simulink model "LUT_liver_pancreas_35"  (R2023b)
settings: Solver=FixedStepAuto  StartTime=0  StopTime=10.1  FixedStep=Timegap  RelTol=1e-3
model workspace (MAT data in the model file):
  T1_input = 1.34
(part 1 of 3)
settings Model: Creator=ppxmr2  LastModifiedBy=ppxmr2

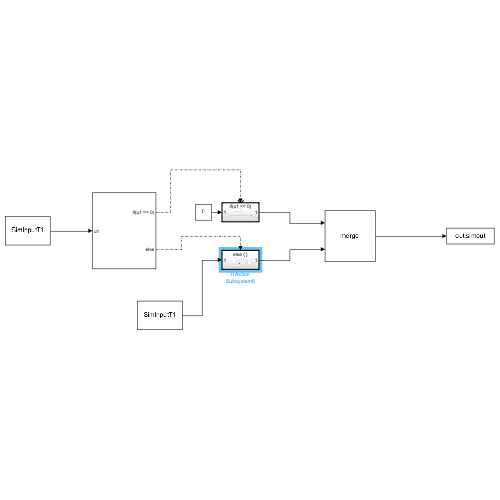
[thumbnail: Simulink's stored preview of the top-level diagram]
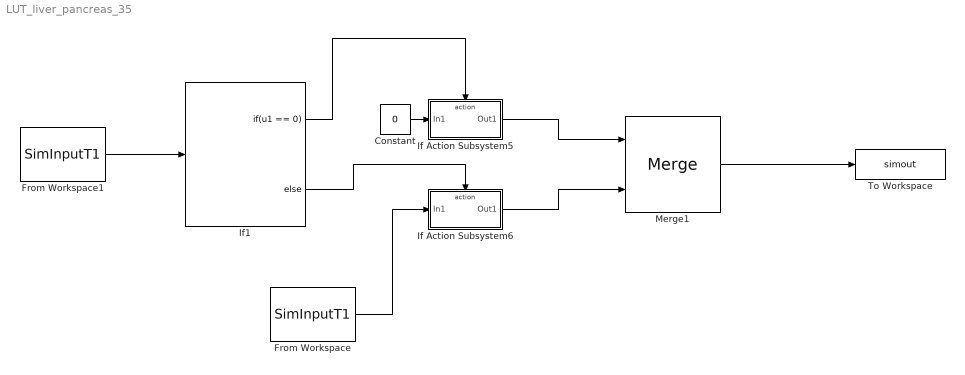
== system LUT_liver_pancreas_35 ==
  Constant : Constant  Value=0
  From Workspace : FromWorkspace  VariableName=SimInputT1  Interpolate=off  OutputAfterFinalValue=Setting to zero
  From Workspace1 : FromWorkspace  VariableName=SimInputT1  Interpolate=off  OutputAfterFinalValue=Setting to zero
  If Action Subsystem5 : Subsystem  TreatAsAtomicUnit=on
  If Action Subsystem6 : Subsystem  TreatAsAtomicUnit=on
  If1 : If  IfExpression=u1 == 0
  Merge1 : Merge
  To Workspace : ToWorkspace  VariableName=simout
  wires:
  From Workspace1/1 -> If1/1
  If1/1 -> If Action Subsystem5/Action
  If1/2 -> If Action Subsystem6/Action
  Constant/1 -> If Action Subsystem5/1(In1)
  If Action Subsystem5/1(Out1) -> Merge1/1
  If Action Subsystem6/1(Out1) -> Merge1/2
  Merge1/1 -> To Workspace/1
  From Workspace/1 -> If Action Subsystem6/1(In1)

== system LUT_liver_pancreas_35/If Action Subsystem5 ==
  In1 : Inport
  Action Port : ActionPort  ActionPortLabel=if(u1 == 0)
  Out1 : Outport
  wires:
  In1/1 -> Out1/1

== system LUT_liver_pancreas_35/If Action Subsystem6 ==
  In1 : Inport
  Action Port : ActionPort  ActionPortLabel=else
  From Workspace1 : FromWorkspace  VariableName=SimInputHR  Interpolate=off  OutputAfterFinalValue=Setting to zero
  If : If  IfExpression=u1 >= 1.495  ElseIfExpressions=u1 >= 0.995
  If Action Subsystem1 : Subsystem  TreatAsAtomicUnit=on
  If Action Subsystem2 : Subsystem  TreatAsAtomicUnit=on
  If Action Subsystem3 : Subsystem  TreatAsAtomicUnit=on
  Merge : Merge  Inputs=3
  Out1 : Outport
  wires:
  Merge/1 -> Out1/1
  From Workspace1/1 -> If/1
  If Action Subsystem1/1(Out1) -> Merge/2
  If Action Subsystem3/1(Out1) -> Merge/3
  In1/1 -> If Action Subsystem2/1(In1), If Action Subsystem1/1(In1), If Action Subsystem3/1(In1)
  If/1 -> If Action Subsystem2/Action
  If/2 -> If Action Subsystem1/Action
  If/3 -> If Action Subsystem3/Action
  If Action Subsystem2/1(Out1) -> Merge/1

== system LUT_liver_pancreas_35/If Action Subsystem6/If Action Subsystem1 ==
  In1 : Inport
  Action Port : ActionPort  ActionPortLabel=elseif(u1 >= 0.995)
  From Workspace2 : FromWorkspace  VariableName=SimInputHR  Interpolate=off  OutputAfterFinalValue=Setting to zero
  If Action Subsystem5 : Subsystem  TreatAsAtomicUnit=on
  If Action Subsystem6 : Subsystem  TreatAsAtomicUnit=on
  If Action Subsystem7 : Subsystem  TreatAsAtomicUnit=on
  If Action Subsystem8 : Subsystem  TreatAsAtomicUnit=on
  If Action Subsystem9 : Subsystem  TreatAsAtomicUnit=on
  If1 : If  IfExpression=u1 >= 1.395  ElseIfExpressions=u1 >= 1.295, u1 >= 1.195, u1 >= 1.095
  Merge1 : Merge  Inputs=5
  Out1 : Outport
  wires:
  In1/1 -> If Action Subsystem7/1(In2), If Action Subsystem8/1(In1), If Action Subsystem9/1(In1), If Action Subsystem5/1(In1), If Action Subsystem6/1(In1)
  From Workspace2/1 -> If1/1
  If Action Subsystem9/1(Out1) -> Merge1/1
  If Action Subsystem6/1(Out1) -> Merge1/5
  If Action Subsystem8/1(Out1) -> Merge1/2
  If Action Subsystem5/1(Out1) -> Merge1/4
  If1/4 -> If Action Subsystem5/Action
  If1/2 -> If Action Subsystem8/Action
  If1/3 -> If Action Subsystem7/Action
  If Action Subsystem7/1(Out2) -> Merge1/3
  If1/5 -> If Action Subsystem6/Action
  If1/1 -> If Action Subsystem9/Action
  Merge1/1 -> Out1/1

== system LUT_liver_pancreas_35/If Action Subsystem6/If Action Subsystem2 ==
  In1 : Inport
  Action Port : ActionPort  ActionPortLabel=if(u1 >= 1.495)
  From Workspace2 : FromWorkspace  VariableName=SimInputHR  Interpolate=off  OutputAfterFinalValue=Setting to zero
  If Action Subsystem5 : Subsystem  TreatAsAtomicUnit=on
  If Action Subsystem6 : Subsystem  TreatAsAtomicUnit=on
  If Action Subsystem7 : Subsystem  TreatAsAtomicUnit=on
  If Action Subsystem8 : Subsystem  TreatAsAtomicUnit=on
  If Action Subsystem9 : Subsystem  TreatAsAtomicUnit=on
  If1 : If  IfExpression=u1 >= 1.895  ElseIfExpressions=u1 >= 1.795, u1 >= 1.695, u1 >= 1.595
  Merge1 : Merge  Inputs=5
  Out1 : Outport
  wires:
  In1/1 -> If Action Subsystem9/1(In1), If Action Subsystem8/1(In1), If Action Subsystem7/1(In1), If Action Subsystem5/1(In1), If Action Subsystem6/1(In1)
  From Workspace2/1 -> If1/1
  If Action Subsystem9/1(Out1) -> Merge1/1
  If1/4 -> If Action Subsystem5/Action
  If1/2 -> If Action Subsystem8/Action
  If1/3 -> If Action Subsystem7/Action
  If1/5 -> If Action Subsystem6/Action
  If1/1 -> If Action Subsystem9/Action
  Merge1/1 -> Out1/1
  If Action Subsystem8/1(Out1) -> Merge1/2
  If Action Subsystem7/1(Out1) -> Merge1/3
  If Action Subsystem6/1(Out1) -> Merge1/5
  If Action Subsystem5/1(Out1) -> Merge1/4

== system LUT_liver_pancreas_35/If Action Subsystem6/If Action Subsystem3 ==
  In1 : Inport
  Action Port : ActionPort  ActionPortLabel=else
  From Workspace2 : FromWorkspace  VariableName=SimInputHR  Interpolate=off  OutputAfterFinalValue=Setting to zero
  If Action Subsystem5 : Subsystem  TreatAsAtomicUnit=on
  If Action Subsystem6 : Subsystem  TreatAsAtomicUnit=on
  If Action Subsystem7 : Subsystem  TreatAsAtomicUnit=on
  If Action Subsystem8 : Subsystem  TreatAsAtomicUnit=on
  If Action Subsystem9 : Subsystem  TreatAsAtomicUnit=on
  If1 : If  IfExpression=u1 >= 0.895  ElseIfExpressions=u1 >= 0.795, u1 >= 0.695, u1 >= 0595
  Merge1 : Merge  Inputs=5
  Out1 : Outport
  wires:
  In1/1 -> If Action Subsystem8/1(In1), If Action Subsystem9/1(In2), If Action Subsystem7/1(In1), If Action Subsystem5/1(In1), If Action Subsystem6/1(In1)
  From Workspace2/1 -> If1/1
  If Action Subsystem9/1(Out2) -> Merge1/1
  If Action Subsystem6/1(Out1) -> Merge1/5
  If Action Subsystem8/1(Out1) -> Merge1/2
  If Action Subsystem5/1(Out1) -> Merge1/4
  If1/4 -> If Action Subsystem5/Action
  If1/2 -> If Action Subsystem8/Action
  If1/3 -> If Action Subsystem7/Action
  If Action Subsystem7/1(Out1) -> Merge1/3
  If1/5 -> If Action Subsystem6/Action
  If1/1 -> If Action Subsystem9/Action
  Merge1/1 -> Out1/1

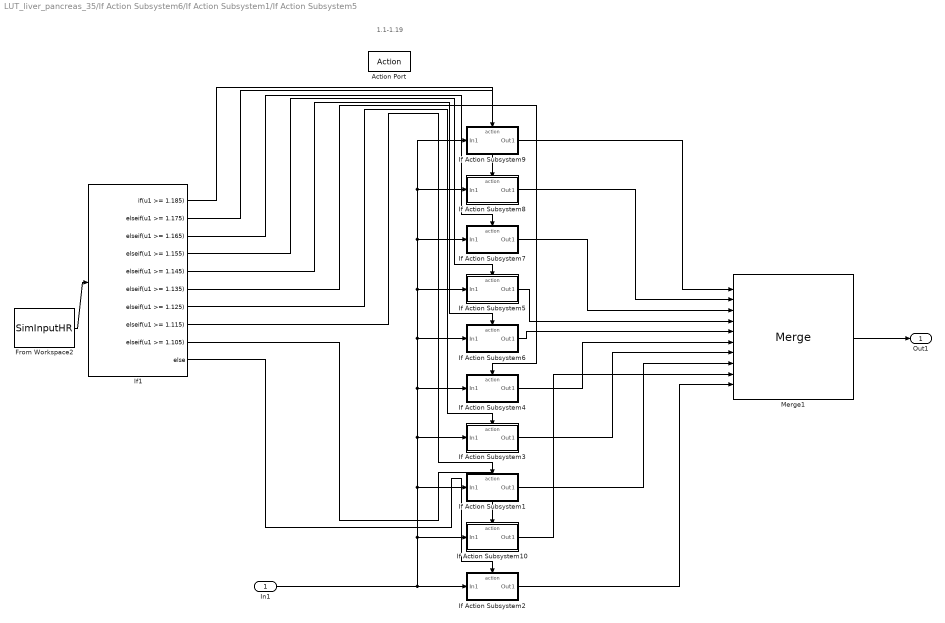
== system LUT_liver_pancreas_35/If Action Subsystem6/If Action Subsystem1/If Action Subsystem5 ==
  note: 1.1-1.19
  In1 : Inport
  Action Port : ActionPort  ActionPortLabel=elseif( u1 >= 1.095)
  From Workspace2 : FromWorkspace  VariableName=SimInputHR  Interpolate=off  OutputAfterFinalValue=Setting to zero
  If Action Subsystem1 : Subsystem  TreatAsAtomicUnit=on
  If Action Subsystem10 : Subsystem  TreatAsAtomicUnit=on
  If Action Subsystem2 : Subsystem  TreatAsAtomicUnit=on
  If Action Subsystem3 : Subsystem  TreatAsAtomicUnit=on
  If Action Subsystem4 : Subsystem  TreatAsAtomicUnit=on
  If Action Subsystem5 : Subsystem  TreatAsAtomicUnit=on
  If Action Subsystem6 : Subsystem  TreatAsAtomicUnit=on
  If Action Subsystem7 : Subsystem  TreatAsAtomicUnit=on
  If Action Subsystem8 : Subsystem  TreatAsAtomicUnit=on
  If Action Subsystem9 : Subsystem  TreatAsAtomicUnit=on
  If1 : If  IfExpression=u1 >= 1.185  ElseIfExpressions=u1 >= 1.175, u1 >= 1.165, u1 >= 1.155, u1 >= 1.145, u1 >= 1.135, u1 >= 1.125, u1 >= 1.115, u1 >= 1.105
  Merge1 : Merge  Inputs=10
  Out1 : Outport
  wires:
  If1/10 -> If Action Subsystem2/Action
  If Action Subsystem4/1(Out1) -> Merge1/6
  From Workspace2/1 -> If1/1
  If Action Subsystem6/1(Out1) -> Merge1/5
  Merge1/1 -> Out1/1
  If1/8 -> If Action Subsystem1/Action
  If Action Subsystem3/1(Out1) -> Merge1/7
  In1/1 -> If Action Subsystem1/1(In1), If Action Subsystem3/1(In1), If Action Subsystem4/1(In1), If Action Subsystem7/1(In1), If Action Subsystem8/1(In1), If Action Subsystem9/1(In1), If Action Subsystem5/1(In1), If Action Subsystem6/1(In1), If Action Subsystem10/1(In1), If Action Subsystem2/1(In1)
  If1/6 -> If Action Subsystem4/Action
  If Action Subsystem1/1(Out1) -> Merge1/8
  If1/4 -> If Action Subsystem5/Action
  If Action Subsystem8/1(Out1) -> Merge1/2
  If1/5 -> If Action Subsystem6/Action
  If Action Subsystem7/1(Out1) -> Merge1/3
  If1/3 -> If Action Subsystem7/Action
  If1/7 -> If Action Subsystem3/Action
  If Action Subsystem5/1(Out1) -> Merge1/4
  If Action Subsystem2/1(Out1) -> Merge1/10
  If1/2 -> If Action Subsystem8/Action
  If1/1 -> If Action Subsystem9/Action
  If Action Subsystem9/1(Out1) -> Merge1/1
  If1/9 -> If Action Subsystem10/Action
  If Action Subsystem10/1(Out1) -> Merge1/9

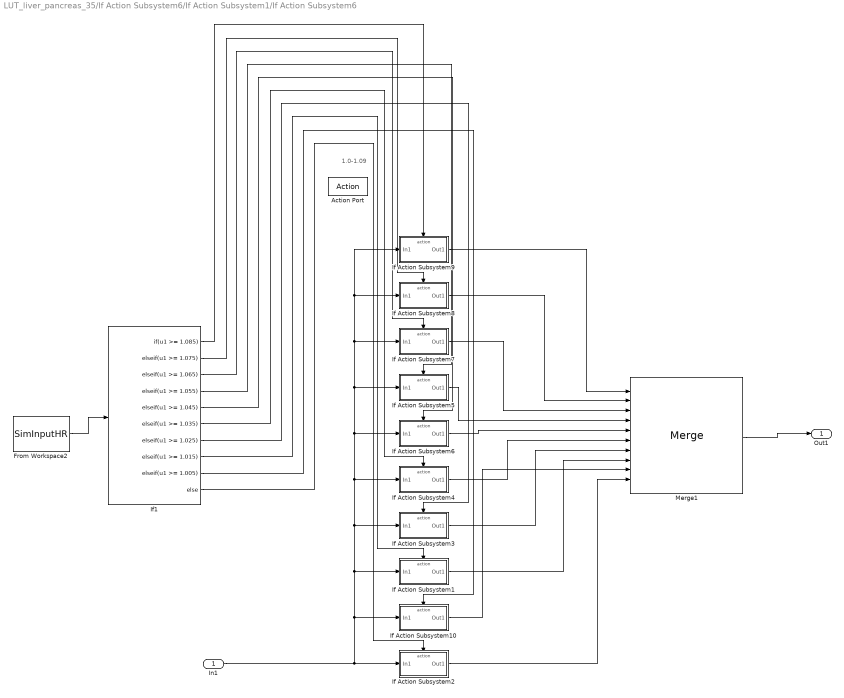
== system LUT_liver_pancreas_35/If Action Subsystem6/If Action Subsystem1/If Action Subsystem6 ==
  note: 1.0-1.09
  In1 : Inport
  Action Port : ActionPort  ActionPortLabel=else
  From Workspace2 : FromWorkspace  VariableName=SimInputHR  Interpolate=off  OutputAfterFinalValue=Setting to zero
  If Action Subsystem1 : Subsystem  TreatAsAtomicUnit=on
  If Action Subsystem10 : Subsystem  TreatAsAtomicUnit=on
  If Action Subsystem2 : Subsystem  TreatAsAtomicUnit=on
  If Action Subsystem3 : Subsystem  TreatAsAtomicUnit=on
  If Action Subsystem4 : Subsystem  TreatAsAtomicUnit=on
  If Action Subsystem5 : Subsystem  TreatAsAtomicUnit=on
  If Action Subsystem6 : Subsystem  TreatAsAtomicUnit=on
  If Action Subsystem7 : Subsystem  TreatAsAtomicUnit=on
  If Action Subsystem8 : Subsystem  TreatAsAtomicUnit=on
  If Action Subsystem9 : Subsystem  TreatAsAtomicUnit=on
  If1 : If  IfExpression=u1 >= 1.085  ElseIfExpressions=u1 >= 1.075, u1 >= 1.065, u1 >= 1.055, u1 >= 1.045, u1 >= 1.035, u1 >= 1.025, u1 >= 1.015, u1 >= 1.005
  Merge1 : Merge  Inputs=10
  Out1 : Outport
  wires:
  If1/10 -> If Action Subsystem2/Action
  If Action Subsystem4/1(Out1) -> Merge1/6
  From Workspace2/1 -> If1/1
  If Action Subsystem6/1(Out1) -> Merge1/5
  Merge1/1 -> Out1/1
  If1/8 -> If Action Subsystem1/Action
  If Action Subsystem3/1(Out1) -> Merge1/7
  In1/1 -> If Action Subsystem1/1(In1), If Action Subsystem3/1(In1), If Action Subsystem4/1(In1), If Action Subsystem7/1(In1), If Action Subsystem8/1(In1), If Action Subsystem9/1(In1), If Action Subsystem5/1(In1), If Action Subsystem6/1(In1), If Action Subsystem10/1(In1), If Action Subsystem2/1(In1)
  If1/6 -> If Action Subsystem4/Action
  If Action Subsystem1/1(Out1) -> Merge1/8
  If1/4 -> If Action Subsystem5/Action
  If Action Subsystem8/1(Out1) -> Merge1/2
  If1/5 -> If Action Subsystem6/Action
  If Action Subsystem7/1(Out1) -> Merge1/3
  If1/3 -> If Action Subsystem7/Action
  If1/7 -> If Action Subsystem3/Action
  If Action Subsystem5/1(Out1) -> Merge1/4
  If Action Subsystem2/1(Out1) -> Merge1/10
  If1/2 -> If Action Subsystem8/Action
  If1/1 -> If Action Subsystem9/Action
  If Action Subsystem9/1(Out1) -> Merge1/1
  If1/9 -> If Action Subsystem10/Action
  If Action Subsystem10/1(Out1) -> Merge1/9

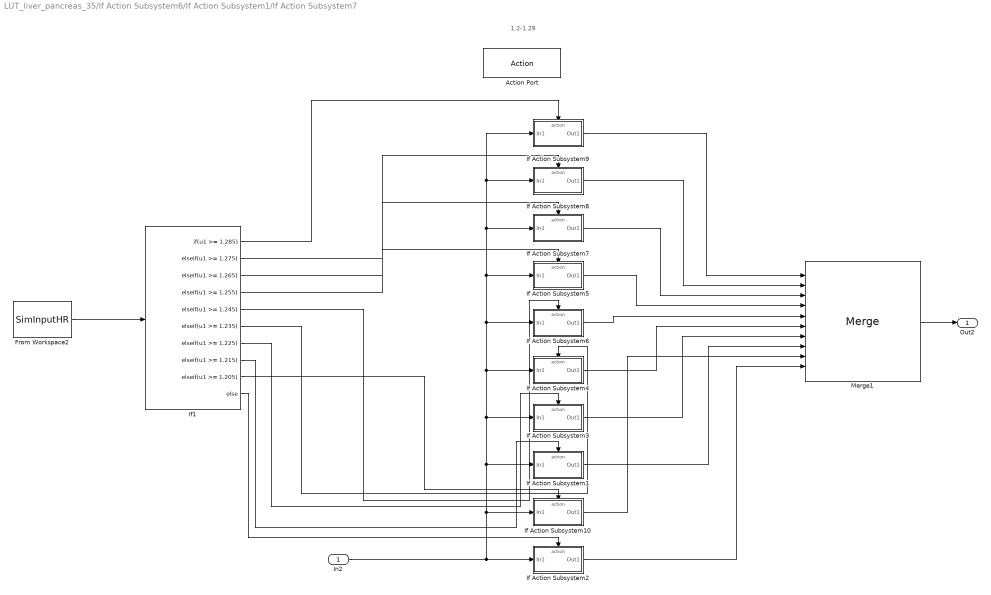
== system LUT_liver_pancreas_35/If Action Subsystem6/If Action Subsystem1/If Action Subsystem7 ==
  note: 1.2-1.29
  In2 : Inport
  Action Port : ActionPort  ActionPortLabel=elseif( u1 >= 1.195)
  From Workspace2 : FromWorkspace  VariableName=SimInputHR  Interpolate=off  OutputAfterFinalValue=Setting to zero
  If Action Subsystem1 : Subsystem  TreatAsAtomicUnit=on
  If Action Subsystem10 : Subsystem  TreatAsAtomicUnit=on
  If Action Subsystem2 : Subsystem  TreatAsAtomicUnit=on
  If Action Subsystem3 : Subsystem  TreatAsAtomicUnit=on
  If Action Subsystem4 : Subsystem  TreatAsAtomicUnit=on
  If Action Subsystem5 : Subsystem  TreatAsAtomicUnit=on
  If Action Subsystem6 : Subsystem  TreatAsAtomicUnit=on
  If Action Subsystem7 : Subsystem  TreatAsAtomicUnit=on
  If Action Subsystem8 : Subsystem  TreatAsAtomicUnit=on
  If Action Subsystem9 : Subsystem  TreatAsAtomicUnit=on
  If1 : If  IfExpression=u1 >= 1.285  ElseIfExpressions=u1 >= 1.275, u1 >= 1.265, u1 >= 1.255, u1 >= 1.245, u1 >= 1.235, u1 >= 1.225, u1 >= 1.215, u1 >= 1.205
  Merge1 : Merge  Inputs=10
  Out2 : Outport
  wires:
  If1/10 -> If Action Subsystem2/Action
  If Action Subsystem4/1(Out1) -> Merge1/6
  From Workspace2/1 -> If1/1
  If Action Subsystem6/1(Out1) -> Merge1/5
  Merge1/1 -> Out2/1
  If1/8 -> If Action Subsystem1/Action
  If Action Subsystem3/1(Out1) -> Merge1/7
  In2/1 -> If Action Subsystem1/1(In1), If Action Subsystem3/1(In1), If Action Subsystem4/1(In1), If Action Subsystem7/1(In1), If Action Subsystem8/1(In1), If Action Subsystem9/1(In1), If Action Subsystem5/1(In1), If Action Subsystem6/1(In1), If Action Subsystem10/1(In1), If Action Subsystem2/1(In1)
  If1/6 -> If Action Subsystem4/Action
  If Action Subsystem1/1(Out1) -> Merge1/8
  If1/4 -> If Action Subsystem5/Action
  If Action Subsystem8/1(Out1) -> Merge1/2
  If1/5 -> If Action Subsystem6/Action
  If Action Subsystem7/1(Out1) -> Merge1/3
  If1/3 -> If Action Subsystem7/Action
  If1/7 -> If Action Subsystem3/Action
  If Action Subsystem5/1(Out1) -> Merge1/4
  If Action Subsystem2/1(Out1) -> Merge1/10
  If1/2 -> If Action Subsystem8/Action
  If1/1 -> If Action Subsystem9/Action
  If Action Subsystem9/1(Out1) -> Merge1/1
  If Action Subsystem10/1(Out1) -> Merge1/9
  If1/9 -> If Action Subsystem10/Action

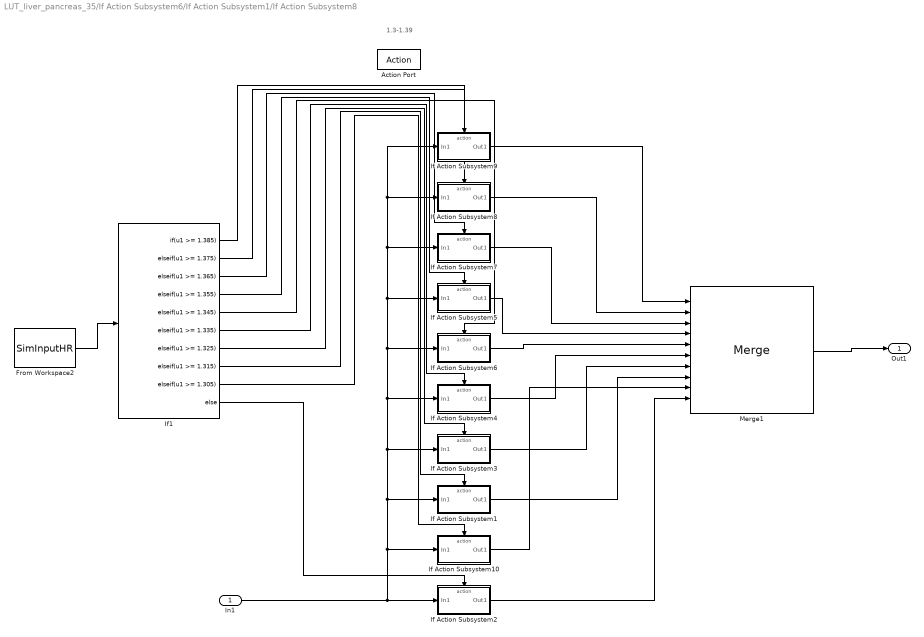
== system LUT_liver_pancreas_35/If Action Subsystem6/If Action Subsystem1/If Action Subsystem8 ==
  note: 1.3-1.39
  In1 : Inport
  Action Port : ActionPort  ActionPortLabel=elseif(u1 >= 1.295)
  From Workspace2 : FromWorkspace  VariableName=SimInputHR  Interpolate=off  OutputAfterFinalValue=Setting to zero
  If Action Subsystem1 : Subsystem  TreatAsAtomicUnit=on
  If Action Subsystem10 : Subsystem  TreatAsAtomicUnit=on
  If Action Subsystem2 : Subsystem  TreatAsAtomicUnit=on
  If Action Subsystem3 : Subsystem  TreatAsAtomicUnit=on
  If Action Subsystem4 : Subsystem  TreatAsAtomicUnit=on
  If Action Subsystem5 : Subsystem  TreatAsAtomicUnit=on
  If Action Subsystem6 : Subsystem  TreatAsAtomicUnit=on
  If Action Subsystem7 : Subsystem  TreatAsAtomicUnit=on
  If Action Subsystem8 : Subsystem  TreatAsAtomicUnit=on
  If Action Subsystem9 : Subsystem  TreatAsAtomicUnit=on
  If1 : If  IfExpression=u1 >= 1.385  ElseIfExpressions=u1 >= 1.375, u1 >= 1.365, u1 >= 1.355, u1 >= 1.345, u1 >= 1.335, u1 >= 1.325, u1 >= 1.315, u1 >= 1.305
  Merge1 : Merge  Inputs=10
  Out1 : Outport
  wires:
  If1/10 -> If Action Subsystem2/Action
  If Action Subsystem4/1(Out1) -> Merge1/6
  From Workspace2/1 -> If1/1
  If Action Subsystem6/1(Out1) -> Merge1/5
  Merge1/1 -> Out1/1
  If1/8 -> If Action Subsystem1/Action
  If Action Subsystem3/1(Out1) -> Merge1/7
  In1/1 -> If Action Subsystem1/1(In1), If Action Subsystem3/1(In1), If Action Subsystem4/1(In1), If Action Subsystem7/1(In1), If Action Subsystem8/1(In1), If Action Subsystem9/1(In1), If Action Subsystem5/1(In1), If Action Subsystem6/1(In1), If Action Subsystem10/1(In1), If Action Subsystem2/1(In1)
  If1/6 -> If Action Subsystem4/Action
  If Action Subsystem1/1(Out1) -> Merge1/8
  If1/4 -> If Action Subsystem5/Action
  If Action Subsystem8/1(Out1) -> Merge1/2
  If1/5 -> If Action Subsystem6/Action
  If Action Subsystem7/1(Out1) -> Merge1/3
  If1/3 -> If Action Subsystem7/Action
  If1/7 -> If Action Subsystem3/Action
  If Action Subsystem5/1(Out1) -> Merge1/4
  If Action Subsystem2/1(Out1) -> Merge1/10
  If1/2 -> If Action Subsystem8/Action
  If1/1 -> If Action Subsystem9/Action
  If Action Subsystem9/1(Out1) -> Merge1/1
  If1/9 -> If Action Subsystem10/Action
  If Action Subsystem10/1(Out1) -> Merge1/9

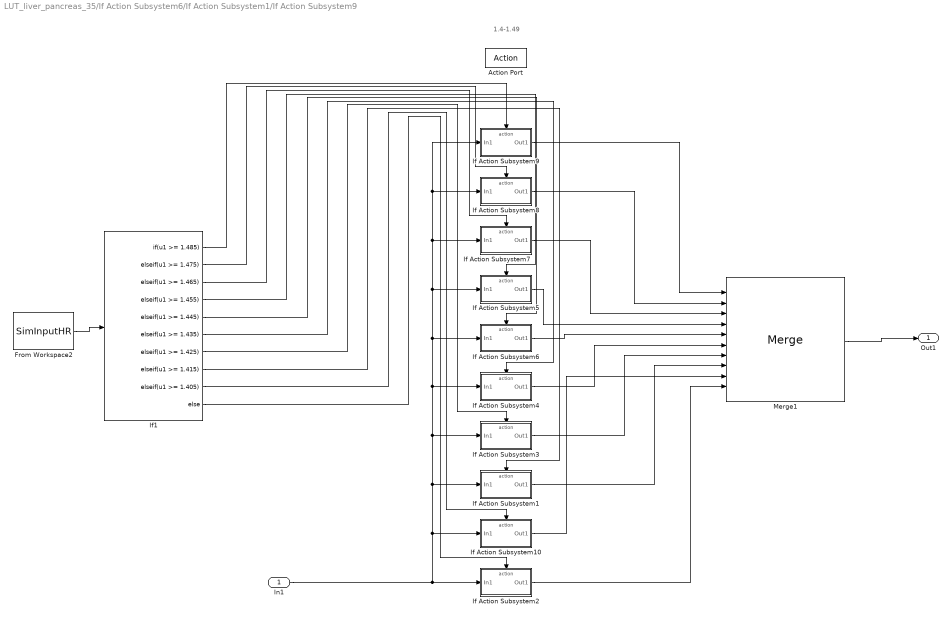
== system LUT_liver_pancreas_35/If Action Subsystem6/If Action Subsystem1/If Action Subsystem9 ==
  note: 1.4-1.49
  In1 : Inport
  Action Port : ActionPort  ActionPortLabel=if(u1 >= 1.395)
  From Workspace2 : FromWorkspace  VariableName=SimInputHR  Interpolate=off  OutputAfterFinalValue=Setting to zero
  If Action Subsystem1 : Subsystem  TreatAsAtomicUnit=on
  If Action Subsystem10 : Subsystem  TreatAsAtomicUnit=on
  If Action Subsystem2 : Subsystem  TreatAsAtomicUnit=on
  If Action Subsystem3 : Subsystem  TreatAsAtomicUnit=on
  If Action Subsystem4 : Subsystem  TreatAsAtomicUnit=on
  If Action Subsystem5 : Subsystem  TreatAsAtomicUnit=on
  If Action Subsystem6 : Subsystem  TreatAsAtomicUnit=on
  If Action Subsystem7 : Subsystem  TreatAsAtomicUnit=on
  If Action Subsystem8 : Subsystem  TreatAsAtomicUnit=on
  If Action Subsystem9 : Subsystem  TreatAsAtomicUnit=on
  If1 : If  IfExpression=u1 >= 1.485  ElseIfExpressions=u1 >= 1.475, u1 >= 1.465, u1 >= 1.455, u1 >= 1.445, u1 >= 1.435, u1 >= 1.425, u1 >= 1.415, u1 >= 1.405
  Merge1 : Merge  Inputs=10
  Out1 : Outport
  wires:
  If1/10 -> If Action Subsystem2/Action
  If Action Subsystem4/1(Out1) -> Merge1/6
  From Workspace2/1 -> If1/1
  If Action Subsystem6/1(Out1) -> Merge1/5
  Merge1/1 -> Out1/1
  If1/8 -> If Action Subsystem1/Action
  If Action Subsystem3/1(Out1) -> Merge1/7
  In1/1 -> If Action Subsystem10/1(In1), If Action Subsystem1/1(In1), If Action Subsystem3/1(In1), If Action Subsystem4/1(In1), If Action Subsystem7/1(In1), If Action Subsystem8/1(In1), If Action Subsystem9/1(In1), If Action Subsystem5/1(In1), If Action Subsystem6/1(In1), If Action Subsystem2/1(In1)
  If1/6 -> If Action Subsystem4/Action
  If Action Subsystem1/1(Out1) -> Merge1/8
  If1/4 -> If Action Subsystem5/Action
  If Action Subsystem8/1(Out1) -> Merge1/2
  If1/5 -> If Action Subsystem6/Action
  If Action Subsystem7/1(Out1) -> Merge1/3
  If1/3 -> If Action Subsystem7/Action
  If1/7 -> If Action Subsystem3/Action
  If Action Subsystem5/1(Out1) -> Merge1/4
  If Action Subsystem2/1(Out1) -> Merge1/10
  If1/2 -> If Action Subsystem8/Action
  If1/1 -> If Action Subsystem9/Action
  If Action Subsystem9/1(Out1) -> Merge1/1
  If1/9 -> If Action Subsystem10/Action
  If Action Subsystem10/1(Out1) -> Merge1/9

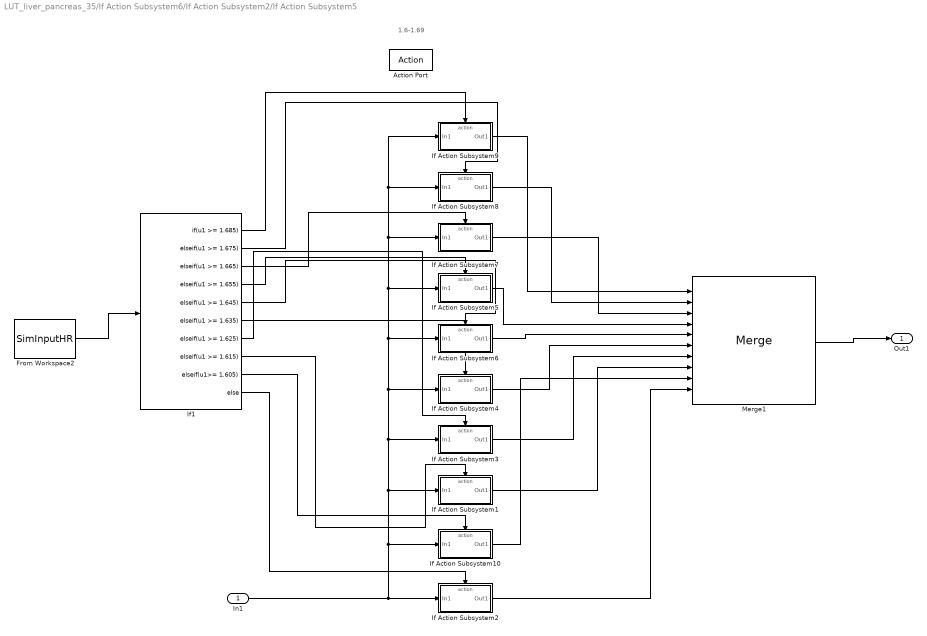
== system LUT_liver_pancreas_35/If Action Subsystem6/If Action Subsystem2/If Action Subsystem5 ==
  note: 1.6-1.69
  In1 : Inport
  Action Port : ActionPort  ActionPortLabel=elseif( u1 >= 1.595)
  From Workspace2 : FromWorkspace  VariableName=SimInputHR  Interpolate=off  OutputAfterFinalValue=Setting to zero
  If Action Subsystem1 : Subsystem  TreatAsAtomicUnit=on
  If Action Subsystem10 : Subsystem  TreatAsAtomicUnit=on
  If Action Subsystem2 : Subsystem  TreatAsAtomicUnit=on
  If Action Subsystem3 : Subsystem  TreatAsAtomicUnit=on
  If Action Subsystem4 : Subsystem  TreatAsAtomicUnit=on
  If Action Subsystem5 : Subsystem  TreatAsAtomicUnit=on
  If Action Subsystem6 : Subsystem  TreatAsAtomicUnit=on
  If Action Subsystem7 : Subsystem  TreatAsAtomicUnit=on
  If Action Subsystem8 : Subsystem  TreatAsAtomicUnit=on
  If Action Subsystem9 : Subsystem  TreatAsAtomicUnit=on
  If1 : If  IfExpression=u1 >= 1.685  ElseIfExpressions=u1 >= 1.675, u1 >= 1.665, u1 >= 1.655, u1 >= 1.645, u1 >= 1.635, u1 >= 1.625, u1 >= 1.615, u1>= 1.605
  Merge1 : Merge  Inputs=10
  Out1 : Outport
  wires:
  If1/2 -> If Action Subsystem8/Action
  If Action Subsystem5/1(Out1) -> Merge1/4
  If1/3 -> If Action Subsystem7/Action
  If Action Subsystem9/1(Out1) -> Merge1/1
  If1/7 -> If Action Subsystem3/Action
  If1/5 -> If Action Subsystem6/Action
  If1/1 -> If Action Subsystem9/Action
  If Action Subsystem4/1(Out1) -> Merge1/6
  If1/10 -> If Action Subsystem2/Action
  If Action Subsystem8/1(Out1) -> Merge1/2
  If1/4 -> If Action Subsystem5/Action
  In1/1 -> If Action Subsystem10/1(In1), If Action Subsystem1/1(In1), If Action Subsystem3/1(In1), If Action Subsystem4/1(In1), If Action Subsystem7/1(In1), If Action Subsystem8/1(In1), If Action Subsystem9/1(In1), If Action Subsystem5/1(In1), If Action Subsystem6/1(In1), If Action Subsystem2/1(In1)
  If Action Subsystem1/1(Out1) -> Merge1/8
  If Action Subsystem2/1(Out1) -> Merge1/10
  If1/8 -> If Action Subsystem1/Action
  If Action Subsystem3/1(Out1) -> Merge1/7
  If1/6 -> If Action Subsystem4/Action
  From Workspace2/1 -> If1/1
  Merge1/1 -> Out1/1
  If Action Subsystem6/1(Out1) -> Merge1/5
  If Action Subsystem7/1(Out1) -> Merge1/3
  If1/9 -> If Action Subsystem10/Action
  If Action Subsystem10/1(Out1) -> Merge1/9

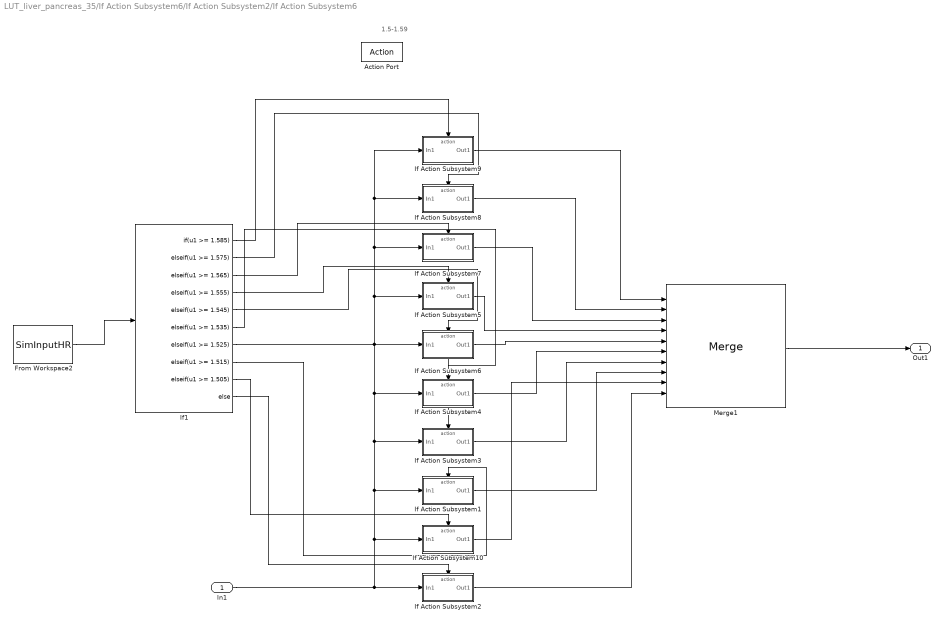
== system LUT_liver_pancreas_35/If Action Subsystem6/If Action Subsystem2/If Action Subsystem6 ==
  note: 1.5-1.59
  In1 : Inport
  Action Port : ActionPort  ActionPortLabel=else
  From Workspace2 : FromWorkspace  VariableName=SimInputHR  Interpolate=off  OutputAfterFinalValue=Setting to zero
  If Action Subsystem1 : Subsystem  TreatAsAtomicUnit=on
  If Action Subsystem10 : Subsystem  TreatAsAtomicUnit=on
  If Action Subsystem2 : Subsystem  TreatAsAtomicUnit=on
  If Action Subsystem3 : Subsystem  TreatAsAtomicUnit=on
  If Action Subsystem4 : Subsystem  TreatAsAtomicUnit=on
  If Action Subsystem5 : Subsystem  TreatAsAtomicUnit=on
  If Action Subsystem6 : Subsystem  TreatAsAtomicUnit=on
  If Action Subsystem7 : Subsystem  TreatAsAtomicUnit=on
  If Action Subsystem8 : Subsystem  TreatAsAtomicUnit=on
  If Action Subsystem9 : Subsystem  TreatAsAtomicUnit=on
  If1 : If  IfExpression=u1 >= 1.585  ElseIfExpressions=u1 >= 1.575, u1 >= 1.565, u1 >= 1.555, u1 >= 1.545, u1 >= 1.535, u1 >= 1.525, u1 >= 1.515, u1 >= 1.505
  Merge1 : Merge  Inputs=10
  Out1 : Outport
  wires:
  If1/2 -> If Action Subsystem8/Action
  If Action Subsystem5/1(Out1) -> Merge1/4
  If1/3 -> If Action Subsystem7/Action
  If Action Subsystem9/1(Out1) -> Merge1/1
  If1/7 -> If Action Subsystem3/Action
  If1/5 -> If Action Subsystem6/Action
  If1/1 -> If Action Subsystem9/Action
  If Action Subsystem4/1(Out1) -> Merge1/6
  If1/10 -> If Action Subsystem2/Action
  If Action Subsystem8/1(Out1) -> Merge1/2
  If1/4 -> If Action Subsystem5/Action
  In1/1 -> If Action Subsystem10/1(In1), If Action Subsystem1/1(In1), If Action Subsystem3/1(In1), If Action Subsystem4/1(In1), If Action Subsystem7/1(In1), If Action Subsystem8/1(In1), If Action Subsystem9/1(In1), If Action Subsystem5/1(In1), If Action Subsystem6/1(In1), If Action Subsystem2/1(In1)
  If Action Subsystem1/1(Out1) -> Merge1/8
  If Action Subsystem2/1(Out1) -> Merge1/10
  If1/8 -> If Action Subsystem1/Action
  If Action Subsystem3/1(Out1) -> Merge1/7
  If1/6 -> If Action Subsystem4/Action
  From Workspace2/1 -> If1/1
  Merge1/1 -> Out1/1
  If Action Subsystem6/1(Out1) -> Merge1/5
  If Action Subsystem7/1(Out1) -> Merge1/3
  If1/9 -> If Action Subsystem10/Action
  If Action Subsystem10/1(Out1) -> Merge1/9

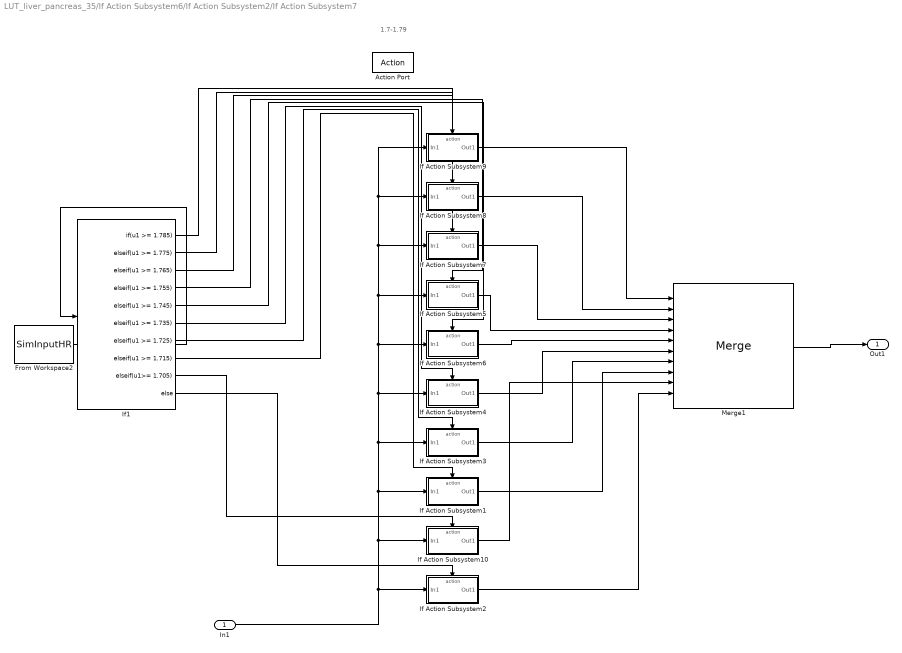
== system LUT_liver_pancreas_35/If Action Subsystem6/If Action Subsystem2/If Action Subsystem7 ==
  note: 1.7-1.79
  In1 : Inport
  Action Port : ActionPort  ActionPortLabel=elseif( u1 >= 1.695)
  From Workspace2 : FromWorkspace  VariableName=SimInputHR  Interpolate=off  OutputAfterFinalValue=Setting to zero
  If Action Subsystem1 : Subsystem  TreatAsAtomicUnit=on
  If Action Subsystem10 : Subsystem  TreatAsAtomicUnit=on
  If Action Subsystem2 : Subsystem  TreatAsAtomicUnit=on
  If Action Subsystem3 : Subsystem  TreatAsAtomicUnit=on
  If Action Subsystem4 : Subsystem  TreatAsAtomicUnit=on
  If Action Subsystem5 : Subsystem  TreatAsAtomicUnit=on
  If Action Subsystem6 : Subsystem  TreatAsAtomicUnit=on
  If Action Subsystem7 : Subsystem  TreatAsAtomicUnit=on
  If Action Subsystem8 : Subsystem  TreatAsAtomicUnit=on
  If Action Subsystem9 : Subsystem  TreatAsAtomicUnit=on
  If1 : If  IfExpression=u1 >= 1.785  ElseIfExpressions=u1 >= 1.775, u1 >= 1.765, u1 >= 1.755, u1 >= 1.745, u1 >= 1.735, u1 >= 1.725, u1 >= 1.715, u1>= 1.705
  Merge1 : Merge  Inputs=10
  Out1 : Outport
  wires:
  If1/2 -> If Action Subsystem8/Action
  If Action Subsystem5/1(Out1) -> Merge1/4
  If1/3 -> If Action Subsystem7/Action
  If Action Subsystem9/1(Out1) -> Merge1/1
  If1/7 -> If Action Subsystem3/Action
  If1/5 -> If Action Subsystem6/Action
  If1/1 -> If Action Subsystem9/Action
  If Action Subsystem4/1(Out1) -> Merge1/6
  If1/10 -> If Action Subsystem2/Action
  If Action Subsystem8/1(Out1) -> Merge1/2
  If1/4 -> If Action Subsystem5/Action
  In1/1 -> If Action Subsystem10/1(In1), If Action Subsystem1/1(In1), If Action Subsystem3/1(In1), If Action Subsystem4/1(In1), If Action Subsystem7/1(In1), If Action Subsystem8/1(In1), If Action Subsystem9/1(In1), If Action Subsystem5/1(In1), If Action Subsystem6/1(In1), If Action Subsystem2/1(In1)
  If Action Subsystem1/1(Out1) -> Merge1/8
  If Action Subsystem2/1(Out1) -> Merge1/10
  If1/8 -> If Action Subsystem1/Action
  If Action Subsystem3/1(Out1) -> Merge1/7
  If1/6 -> If Action Subsystem4/Action
  From Workspace2/1 -> If1/1
  Merge1/1 -> Out1/1
  If Action Subsystem6/1(Out1) -> Merge1/5
  If Action Subsystem7/1(Out1) -> Merge1/3
  If Action Subsystem10/1(Out1) -> Merge1/9
  If1/9 -> If Action Subsystem10/Action

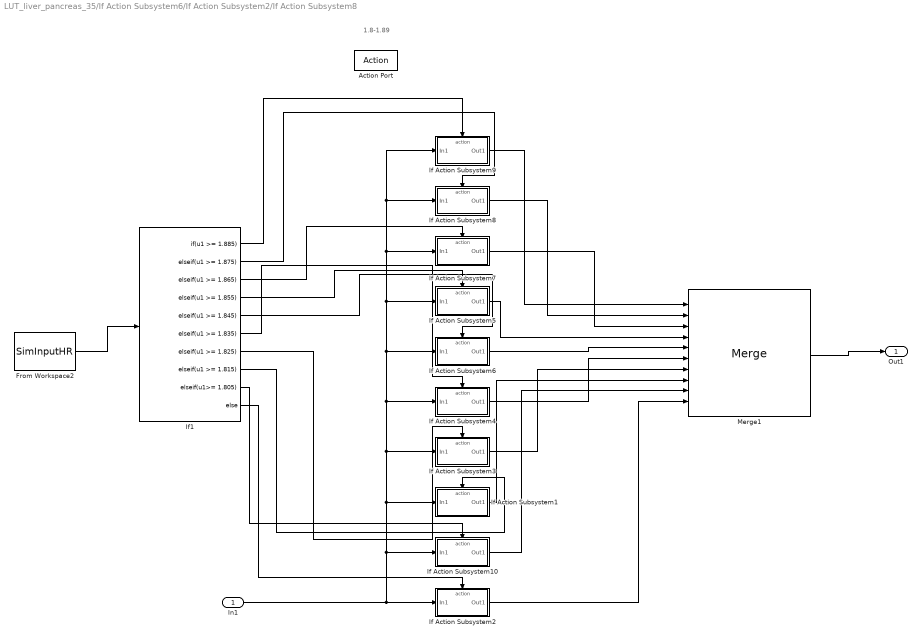
== system LUT_liver_pancreas_35/If Action Subsystem6/If Action Subsystem2/If Action Subsystem8 ==
  note: 1.8-1.89
  In1 : Inport
  Action Port : ActionPort  ActionPortLabel=elseif(u1 >= 1.795)
  From Workspace2 : FromWorkspace  VariableName=SimInputHR  Interpolate=off  OutputAfterFinalValue=Setting to zero
  If Action Subsystem1 : Subsystem  TreatAsAtomicUnit=on
  If Action Subsystem10 : Subsystem  TreatAsAtomicUnit=on
  If Action Subsystem2 : Subsystem  TreatAsAtomicUnit=on
  If Action Subsystem3 : Subsystem  TreatAsAtomicUnit=on
  If Action Subsystem4 : Subsystem  TreatAsAtomicUnit=on
  If Action Subsystem5 : Subsystem  TreatAsAtomicUnit=on
  If Action Subsystem6 : Subsystem  TreatAsAtomicUnit=on
  If Action Subsystem7 : Subsystem  TreatAsAtomicUnit=on
  If Action Subsystem8 : Subsystem  TreatAsAtomicUnit=on
  If Action Subsystem9 : Subsystem  TreatAsAtomicUnit=on
  If1 : If  IfExpression=u1 >= 1.885  ElseIfExpressions=u1 >= 1.875, u1 >= 1.865, u1 >= 1.855, u1 >= 1.845, u1 >= 1.835, u1 >= 1.825, u1 >= 1.815, u1>= 1.805
  Merge1 : Merge  Inputs=10
  Out1 : Outport
  wires:
  If1/2 -> If Action Subsystem8/Action
  If Action Subsystem5/1(Out1) -> Merge1/4
  If1/3 -> If Action Subsystem7/Action
  If Action Subsystem9/1(Out1) -> Merge1/1
  If1/7 -> If Action Subsystem3/Action
  If1/5 -> If Action Subsystem6/Action
  If1/1 -> If Action Subsystem9/Action
  If Action Subsystem4/1(Out1) -> Merge1/6
  If1/10 -> If Action Subsystem2/Action
  If Action Subsystem8/1(Out1) -> Merge1/2
  If1/4 -> If Action Subsystem5/Action
  In1/1 -> If Action Subsystem10/1(In1), If Action Subsystem1/1(In1), If Action Subsystem3/1(In1), If Action Subsystem4/1(In1), If Action Subsystem7/1(In1), If Action Subsystem8/1(In1), If Action Subsystem9/1(In1), If Action Subsystem5/1(In1), If Action Subsystem6/1(In1), If Action Subsystem2/1(In1)
  If Action Subsystem1/1(Out1) -> Merge1/8
  If Action Subsystem2/1(Out1) -> Merge1/10
  If1/8 -> If Action Subsystem1/Action
  If Action Subsystem3/1(Out1) -> Merge1/7
  If1/6 -> If Action Subsystem4/Action
  From Workspace2/1 -> If1/1
  Merge1/1 -> Out1/1
  If Action Subsystem6/1(Out1) -> Merge1/5
  If Action Subsystem7/1(Out1) -> Merge1/3
  If1/9 -> If Action Subsystem10/Action
  If Action Subsystem10/1(Out1) -> Merge1/9

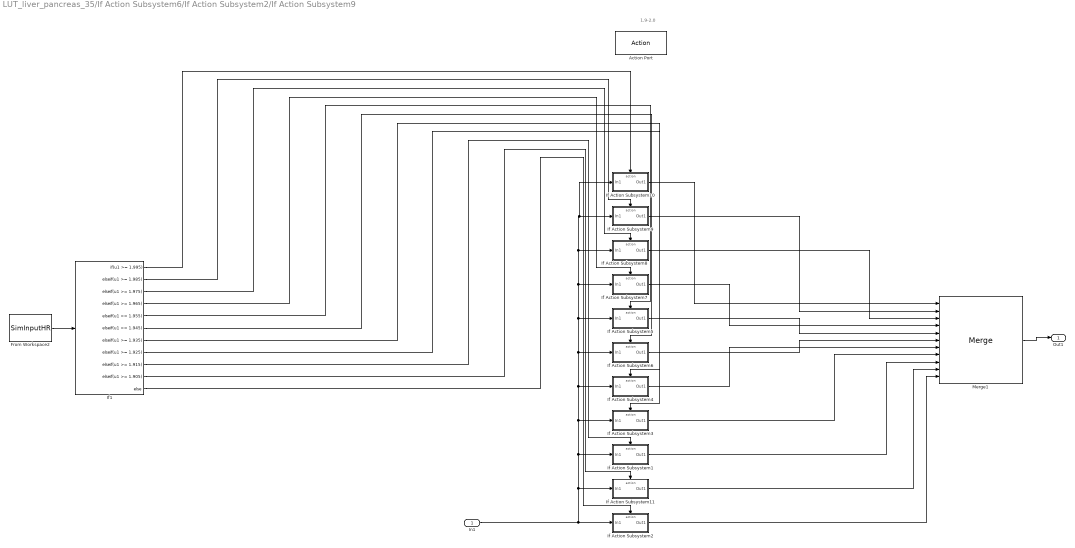
== system LUT_liver_pancreas_35/If Action Subsystem6/If Action Subsystem2/If Action Subsystem9 ==
  note: 1.9-2.0
  In1 : Inport
  Action Port : ActionPort  ActionPortLabel=if(u1 >= 1.895)
  From Workspace2 : FromWorkspace  VariableName=SimInputHR  Interpolate=off  OutputAfterFinalValue=Setting to zero
  If Action Subsystem1 : Subsystem  TreatAsAtomicUnit=on
  If Action Subsystem10 : Subsystem  TreatAsAtomicUnit=on
  If Action Subsystem11 : Subsystem  TreatAsAtomicUnit=on
  If Action Subsystem2 : Subsystem  TreatAsAtomicUnit=on
  If Action Subsystem3 : Subsystem  TreatAsAtomicUnit=on
  If Action Subsystem4 : Subsystem  TreatAsAtomicUnit=on
  If Action Subsystem5 : Subsystem  TreatAsAtomicUnit=on
  If Action Subsystem6 : Subsystem  TreatAsAtomicUnit=on
  If Action Subsystem7 : Subsystem  TreatAsAtomicUnit=on
  If Action Subsystem8 : Subsystem  TreatAsAtomicUnit=on
  If Action Subsystem9 : Subsystem  TreatAsAtomicUnit=on
  If1 : If  IfExpression=u1 >= 1.995  ElseIfExpressions=u1 >= 1.985, u1 >= 1.975, u1 >= 1.965, u1 >= 1.955, u1 >= 1.945, u1 >= 1.935, u1 >= 1.925, u1 >= 1.915, u1 >= 1.905
  Merge1 : Merge  Inputs=11
  Out1 : Outport
  wires:
  Merge1/1 -> Out1/1
  From Workspace2/1 -> If1/1
  If1/2 -> If Action Subsystem9/Action
  If1/3 -> If Action Subsystem8/Action
  If1/4 -> If Action Subsystem7/Action
  If1/5 -> If Action Subsystem5/Action
  If1/6 -> If Action Subsystem6/Action
  If1/7 -> If Action Subsystem4/Action
  If1/8 -> If Action Subsystem3/Action
  If1/9 -> If Action Subsystem1/Action
  If1/11 -> If Action Subsystem2/Action
  If Action Subsystem9/1(Out1) -> Merge1/2
  If Action Subsystem8/1(Out1) -> Merge1/3
  If Action Subsystem7/1(Out1) -> Merge1/4
  If Action Subsystem5/1(Out1) -> Merge1/5
  If Action Subsystem6/1(Out1) -> Merge1/6
  If Action Subsystem4/1(Out1) -> Merge1/7
  If Action Subsystem3/1(Out1) -> Merge1/8
  If Action Subsystem2/1(Out1) -> Merge1/11
  If Action Subsystem1/1(Out1) -> Merge1/9
  In1/1 -> If Action Subsystem1/1(In1), If Action Subsystem3/1(In1), If Action Subsystem4/1(In1), If Action Subsystem7/1(In1), If Action Subsystem8/1(In1), If Action Subsystem10/1(In1), If Action Subsystem9/1(In1), If Action Subsystem5/1(In1), If Action Subsystem6/1(In1), If Action Subsystem11/1(In1), If Action Subsystem2/1(In1)
  If1/1 -> If Action Subsystem10/Action
  If Action Subsystem10/1(Out1) -> Merge1/1
  If1/10 -> If Action Subsystem11/Action
  If Action Subsystem11/1(Out1) -> Merge1/10

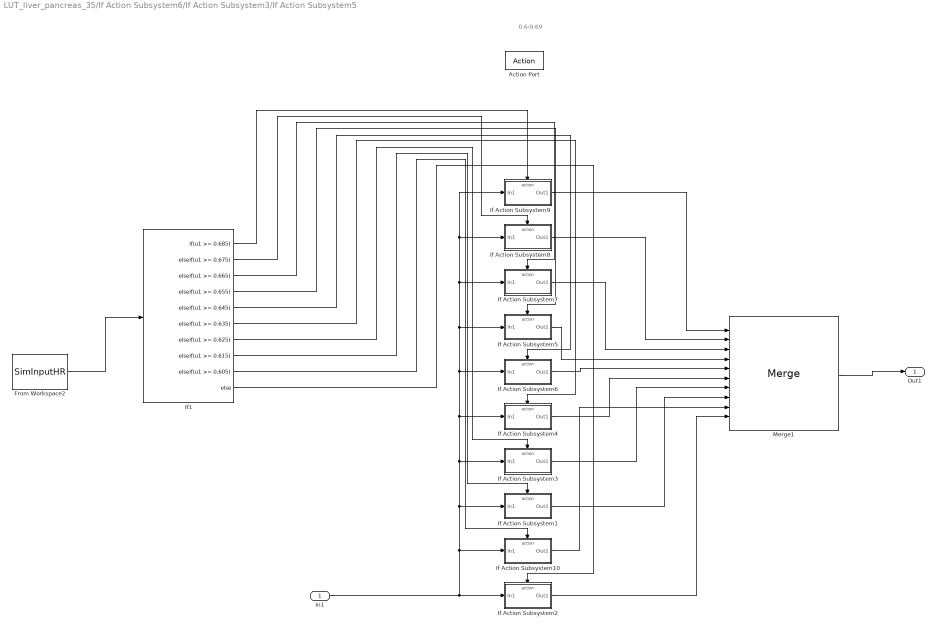
== system LUT_liver_pancreas_35/If Action Subsystem6/If Action Subsystem3/If Action Subsystem5 ==
  note: 0.6-0.69
  In1 : Inport
  Action Port : ActionPort  ActionPortLabel=elseif( u1 >= 0595)
  From Workspace2 : FromWorkspace  VariableName=SimInputHR  Interpolate=off  OutputAfterFinalValue=Setting to zero
  If Action Subsystem1 : Subsystem  TreatAsAtomicUnit=on
  If Action Subsystem10 : Subsystem  TreatAsAtomicUnit=on
  If Action Subsystem2 : Subsystem  TreatAsAtomicUnit=on
  If Action Subsystem3 : Subsystem  TreatAsAtomicUnit=on
  If Action Subsystem4 : Subsystem  TreatAsAtomicUnit=on
  If Action Subsystem5 : Subsystem  TreatAsAtomicUnit=on
  If Action Subsystem6 : Subsystem  TreatAsAtomicUnit=on
  If Action Subsystem7 : Subsystem  TreatAsAtomicUnit=on
  If Action Subsystem8 : Subsystem  TreatAsAtomicUnit=on
  If Action Subsystem9 : Subsystem  TreatAsAtomicUnit=on
  If1 : If  IfExpression=u1 >= 0.685  ElseIfExpressions=u1 >= 0.675, u1 >= 0.665, u1 >= 0.655, u1 >= 0.645, u1 >= 0.635, u1 >= 0.625, u1 >= 0.615, u1 >= 0.605
  Merge1 : Merge  Inputs=10
  Out1 : Outport
  wires:
  If1/10 -> If Action Subsystem2/Action
  If Action Subsystem4/1(Out1) -> Merge1/6
  From Workspace2/1 -> If1/1
  If Action Subsystem6/1(Out1) -> Merge1/5
  Merge1/1 -> Out1/1
  If1/8 -> If Action Subsystem1/Action
  If Action Subsystem3/1(Out1) -> Merge1/7
  In1/1 -> If Action Subsystem1/1(In1), If Action Subsystem3/1(In1), If Action Subsystem4/1(In1), If Action Subsystem7/1(In1), If Action Subsystem8/1(In1), If Action Subsystem9/1(In1), If Action Subsystem5/1(In1), If Action Subsystem6/1(In1), If Action Subsystem10/1(In1), If Action Subsystem2/1(In1)
  If1/6 -> If Action Subsystem4/Action
  If Action Subsystem1/1(Out1) -> Merge1/8
  If1/4 -> If Action Subsystem5/Action
  If Action Subsystem8/1(Out1) -> Merge1/2
  If1/5 -> If Action Subsystem6/Action
  If Action Subsystem7/1(Out1) -> Merge1/3
  If1/3 -> If Action Subsystem7/Action
  If1/7 -> If Action Subsystem3/Action
  If Action Subsystem5/1(Out1) -> Merge1/4
  If Action Subsystem2/1(Out1) -> Merge1/10
  If1/2 -> If Action Subsystem8/Action
  If1/1 -> If Action Subsystem9/Action
  If Action Subsystem9/1(Out1) -> Merge1/1
  If Action Subsystem10/1(Out1) -> Merge1/9
  If1/9 -> If Action Subsystem10/Action

== system LUT_liver_pancreas_35/If Action Subsystem6/If Action Subsystem3/If Action Subsystem6 ==
  note: 0.5-0.59
  In1 : Inport
  Action Port : ActionPort  ActionPortLabel=else
  From Workspace2 : FromWorkspace  VariableName=SimInputHR  Interpolate=off  OutputAfterFinalValue=Setting to zero
  If Action Subsystem1 : Subsystem  TreatAsAtomicUnit=on
  If Action Subsystem10 : Subsystem  TreatAsAtomicUnit=on
  If Action Subsystem2 : Subsystem  TreatAsAtomicUnit=on
  If Action Subsystem3 : Subsystem  TreatAsAtomicUnit=on
  If Action Subsystem4 : Subsystem  TreatAsAtomicUnit=on
  If Action Subsystem5 : Subsystem  TreatAsAtomicUnit=on
  If Action Subsystem6 : Subsystem  TreatAsAtomicUnit=on
  If Action Subsystem7 : Subsystem  TreatAsAtomicUnit=on
  If Action Subsystem8 : Subsystem  TreatAsAtomicUnit=on
  If Action Subsystem9 : Subsystem  TreatAsAtomicUnit=on
  If1 : If  IfExpression=u1 >= 0.585  ElseIfExpressions=u1 >= 0.575, u1 >= 0.565, u1 >= 0.555, u1 >= 0.545, u1 >= 0.535, u1 >= 0.525, u1 >= 0.515, u1 >= 0.505
  Merge1 : Merge  Inputs=10
  Out1 : Outport
  wires:
  If1/10 -> If Action Subsystem2/Action
  If Action Subsystem4/1(Out1) -> Merge1/6
  From Workspace2/1 -> If1/1
  If Action Subsystem6/1(Out1) -> Merge1/5
  Merge1/1 -> Out1/1
  If1/8 -> If Action Subsystem1/Action
  If Action Subsystem3/1(Out1) -> Merge1/7
  In1/1 -> If Action Subsystem1/1(In1), If Action Subsystem3/1(In1), If Action Subsystem4/1(In1), If Action Subsystem7/1(In1), If Action Subsystem8/1(In1), If Action Subsystem9/1(In1), If Action Subsystem5/1(In1), If Action Subsystem6/1(In1), If Action Subsystem10/1(In1), If Action Subsystem2/1(In1)
  If1/6 -> If Action Subsystem4/Action
  If Action Subsystem1/1(Out1) -> Merge1/8
  If1/4 -> If Action Subsystem5/Action
  If Action Subsystem8/1(Out1) -> Merge1/2
  If1/5 -> If Action Subsystem6/Action
  If Action Subsystem7/1(Out1) -> Merge1/3
  If1/3 -> If Action Subsystem7/Action
  If1/7 -> If Action Subsystem3/Action
  If Action Subsystem5/1(Out1) -> Merge1/4
  If Action Subsystem2/1(Out1) -> Merge1/10
  If1/2 -> If Action Subsystem8/Action
  If1/1 -> If Action Subsystem9/Action
  If Action Subsystem9/1(Out1) -> Merge1/1
  If Action Subsystem10/1(Out1) -> Merge1/9
  If1/9 -> If Action Subsystem10/Action

== system LUT_liver_pancreas_35/If Action Subsystem6/If Action Subsystem3/If Action Subsystem7 ==
  note: 0.7-0.79
  In1 : Inport
  Action Port : ActionPort  ActionPortLabel=elseif( u1 >= 0.695)
  From Workspace2 : FromWorkspace  VariableName=SimInputHR  Interpolate=off  OutputAfterFinalValue=Setting to zero
  If Action Subsystem1 : Subsystem  TreatAsAtomicUnit=on
  If Action Subsystem10 : Subsystem  TreatAsAtomicUnit=on
  If Action Subsystem2 : Subsystem  TreatAsAtomicUnit=on
  If Action Subsystem3 : Subsystem  TreatAsAtomicUnit=on
  If Action Subsystem4 : Subsystem  TreatAsAtomicUnit=on
  If Action Subsystem5 : Subsystem  TreatAsAtomicUnit=on
  If Action Subsystem6 : Subsystem  TreatAsAtomicUnit=on
  If Action Subsystem7 : Subsystem  TreatAsAtomicUnit=on
  If Action Subsystem8 : Subsystem  TreatAsAtomicUnit=on
  If Action Subsystem9 : Subsystem  TreatAsAtomicUnit=on
  If1 : If  IfExpression=u1 >= 0.785  ElseIfExpressions=u1 >= 0.775, u1 >= 0.765, u1 >= 0.755, u1 >= 0.745, u1 >= 0.735, u1 >= 0.725, u1 >= 0.715, u1 >= 0.705
  Merge1 : Merge  Inputs=10
  Out1 : Outport
  wires:
  If1/10 -> If Action Subsystem2/Action
  If Action Subsystem4/1(Out1) -> Merge1/6
  From Workspace2/1 -> If1/1
  If Action Subsystem6/1(Out1) -> Merge1/5
  Merge1/1 -> Out1/1
  If1/8 -> If Action Subsystem1/Action
  If Action Subsystem3/1(Out1) -> Merge1/7
  In1/1 -> If Action Subsystem1/1(In1), If Action Subsystem3/1(In1), If Action Subsystem4/1(In1), If Action Subsystem7/1(In1), If Action Subsystem8/1(In1), If Action Subsystem9/1(In1), If Action Subsystem5/1(In1), If Action Subsystem6/1(In1), If Action Subsystem10/1(In1), If Action Subsystem2/1(In1)
  If1/6 -> If Action Subsystem4/Action
  If Action Subsystem1/1(Out1) -> Merge1/8
  If1/4 -> If Action Subsystem5/Action
  If Action Subsystem8/1(Out1) -> Merge1/2
  If1/5 -> If Action Subsystem6/Action
  If Action Subsystem7/1(Out1) -> Merge1/3
  If1/3 -> If Action Subsystem7/Action
  If1/7 -> If Action Subsystem3/Action
  If Action Subsystem5/1(Out1) -> Merge1/4
  If Action Subsystem2/1(Out1) -> Merge1/10
  If1/2 -> If Action Subsystem8/Action
  If1/1 -> If Action Subsystem9/Action
  If Action Subsystem9/1(Out1) -> Merge1/1
  If1/9 -> If Action Subsystem10/Action
  If Action Subsystem10/1(Out1) -> Merge1/9

== system LUT_liver_pancreas_35/If Action Subsystem6/If Action Subsystem3/If Action Subsystem8 ==
  note: 0.8-0.89
  In1 : Inport
  Action Port : ActionPort  ActionPortLabel=elseif(u1 >= 0.795)
  From Workspace2 : FromWorkspace  VariableName=SimInputHR  Interpolate=off  OutputAfterFinalValue=Setting to zero
  If Action Subsystem1 : Subsystem  TreatAsAtomicUnit=on
  If Action Subsystem10 : Subsystem  TreatAsAtomicUnit=on
  If Action Subsystem2 : Subsystem  TreatAsAtomicUnit=on
  If Action Subsystem3 : Subsystem  TreatAsAtomicUnit=on
  If Action Subsystem4 : Subsystem  TreatAsAtomicUnit=on
  If Action Subsystem5 : Subsystem  TreatAsAtomicUnit=on
  If Action Subsystem6 : Subsystem  TreatAsAtomicUnit=on
  If Action Subsystem7 : Subsystem  TreatAsAtomicUnit=on
  If Action Subsystem8 : Subsystem  TreatAsAtomicUnit=on
  If Action Subsystem9 : Subsystem  TreatAsAtomicUnit=on
  If1 : If  IfExpression=u1 >= 0.885  ElseIfExpressions=u1 >= 0.875, u1 >= 0.865, u1 >= 0.855, u1 >= 0.845, u1 >= 0.835, u1 >= 0.825, u1 >= 0.815, u1 >= 0.805
  Merge1 : Merge  Inputs=10
  Out1 : Outport
  wires:
  If1/10 -> If Action Subsystem2/Action
  If Action Subsystem4/1(Out1) -> Merge1/6
  From Workspace2/1 -> If1/1
  If Action Subsystem6/1(Out1) -> Merge1/5
  Merge1/1 -> Out1/1
  If1/8 -> If Action Subsystem1/Action
  If Action Subsystem3/1(Out1) -> Merge1/7
  In1/1 -> If Action Subsystem1/1(In1), If Action Subsystem3/1(In1), If Action Subsystem4/1(In1), If Action Subsystem7/1(In1), If Action Subsystem8/1(In1), If Action Subsystem9/1(In1), If Action Subsystem5/1(In1), If Action Subsystem6/1(In1), If Action Subsystem10/1(In1), If Action Subsystem2/1(In1)
  If1/6 -> If Action Subsystem4/Action
  If Action Subsystem1/1(Out1) -> Merge1/8
  If1/4 -> If Action Subsystem5/Action
  If Action Subsystem8/1(Out1) -> Merge1/2
  If1/5 -> If Action Subsystem6/Action
  If Action Subsystem7/1(Out1) -> Merge1/3
  If1/3 -> If Action Subsystem7/Action
  If1/7 -> If Action Subsystem3/Action
  If Action Subsystem5/1(Out1) -> Merge1/4
  If Action Subsystem2/1(Out1) -> Merge1/10
  If1/2 -> If Action Subsystem8/Action
  If1/1 -> If Action Subsystem9/Action
  If Action Subsystem9/1(Out1) -> Merge1/1
  If1/9 -> If Action Subsystem10/Action
  If Action Subsystem10/1(Out1) -> Merge1/9

== system LUT_liver_pancreas_35/If Action Subsystem6/If Action Subsystem3/If Action Subsystem9 ==
  note: 0.9-0.99
  In2 : Inport
  Action Port : ActionPort  ActionPortLabel=if(u1 >= 0.895)
  From Workspace2 : FromWorkspace  VariableName=SimInputHR  Interpolate=off  OutputAfterFinalValue=Setting to zero
  If Action Subsystem1 : Subsystem  TreatAsAtomicUnit=on
  If Action Subsystem10 : Subsystem  TreatAsAtomicUnit=on
  If Action Subsystem2 : Subsystem  TreatAsAtomicUnit=on
  If Action Subsystem3 : Subsystem  TreatAsAtomicUnit=on
  If Action Subsystem4 : Subsystem  TreatAsAtomicUnit=on
  If Action Subsystem5 : Subsystem  TreatAsAtomicUnit=on
  If Action Subsystem6 : Subsystem  TreatAsAtomicUnit=on
  If Action Subsystem7 : Subsystem  TreatAsAtomicUnit=on
  If Action Subsystem8 : Subsystem  TreatAsAtomicUnit=on
  If Action Subsystem9 : Subsystem  TreatAsAtomicUnit=on
  If1 : If  IfExpression=u1 >= 0.985  ElseIfExpressions=u1 >= 0.975, u1 >= 0.965, u1 >= 0.955, u1 >= 0.945, u1 >= 0.935, u1 >= 0.925, u1 >= 0.915, u1 >= 0.905
  Merge1 : Merge  Inputs=10
  Out2 : Outport
  wires:
  If1/10 -> If Action Subsystem2/Action
  If Action Subsystem4/1(Out1) -> Merge1/6
  From Workspace2/1 -> If1/1
  If Action Subsystem6/1(Out1) -> Merge1/5
  Merge1/1 -> Out2/1
  If1/8 -> If Action Subsystem1/Action
  If Action Subsystem3/1(Out1) -> Merge1/7
  In2/1 -> If Action Subsystem10/1(In1), If Action Subsystem1/1(In1), If Action Subsystem3/1(In1), If Action Subsystem4/1(In1), If Action Subsystem7/1(In1), If Action Subsystem8/1(In1), If Action Subsystem9/1(In1), If Action Subsystem5/1(In1), If Action Subsystem6/1(In1), If Action Subsystem2/1(In1)
  If1/6 -> If Action Subsystem4/Action
  If Action Subsystem1/1(Out1) -> Merge1/8
  If1/4 -> If Action Subsystem5/Action
  If Action Subsystem8/1(Out1) -> Merge1/2
  If1/5 -> If Action Subsystem6/Action
  If Action Subsystem7/1(Out1) -> Merge1/3
  If1/3 -> If Action Subsystem7/Action
  If1/7 -> If Action Subsystem3/Action
  If Action Subsystem5/1(Out1) -> Merge1/4
  If Action Subsystem2/1(Out1) -> Merge1/10
  If1/2 -> If Action Subsystem8/Action
  If1/1 -> If Action Subsystem9/Action
  If Action Subsystem9/1(Out1) -> Merge1/1
  If1/9 -> If Action Subsystem10/Action
  If Action Subsystem10/1(Out1) -> Merge1/9

== system LUT_liver_pancreas_35/If Action Subsystem6/If Action Subsystem1/If Action Subsystem5/If Action Subsystem1 ==
  In1 : Inport
  Action Port : ActionPort  ActionPortLabel=elseif( u1 >= 1.115)
  LUT 1.12RR : Lookup_n-D  NumberOfTableDimensions=1  BreakpointsForDimension1=[411.6381;552.7409;649.7749;746.6144;843.2954;939.8722;1036.381;1132.843;1229.274;1325.682;1422.074;1518.454;1614.825;1711.188;1807.546;1903.898;2000.247]  Table=[400;500;600;700;800;900;1000;1100;1200;1300;1400;1500;1600;1700;1800;1900;2000]  InternalRulePriority=Speed  RndMeth=Simplest
  Out1 : Outport
  wires:
  In1/1 -> LUT 1.12RR/1
  LUT 1.12RR/1 -> Out1/1

== system LUT_liver_pancreas_35/If Action Subsystem6/If Action Subsystem1/If Action Subsystem5/If Action Subsystem10 ==
  In1 : Inport
  Action Port : ActionPort  ActionPortLabel=elseif( u1 >= 1.105)
  LUT 1.11RR : Lookup_n-D  NumberOfTableDimensions=1  BreakpointsForDimension1=[411.7787;553.0469;650.2021;747.1738;843.994;940.7145;1037.37;1133.981;1230.562;1327.122;1423.666;1520.199;1616.724;1713.241;1809.753;1906.26;2002.763]  Table=[400;500;600;700;800;900;1000;1100;1200;1300;1400;1500;1600;1700;1800;1900;2000]  InternalRulePriority=Speed  RndMeth=Simplest
  Out1 : Outport
  wires:
  In1/1 -> LUT 1.11RR/1
  LUT 1.11RR/1 -> Out1/1

== system LUT_liver_pancreas_35/If Action Subsystem6/If Action Subsystem1/If Action Subsystem5/If Action Subsystem2 ==
  In1 : Inport
  Action Port : ActionPort  ActionPortLabel=else
  LUT 1.10RR : Lookup_n-D  NumberOfTableDimensions=1  BreakpointsForDimension1=[411.9215;553.3602;650.6398;747.7471;844.7096;941.577;1038.382;1135.146;1231.88;1328.595;1425.295;1521.984;1618.665;1715.34;1812.01;1908.675;2005.335]  Table=[400;500;600;700;800;900;1000;1100;1200;1300;1400;1500;1600;1700;1800;1900;2000]  InternalRulePriority=Speed  RndMeth=Simplest
  Out1 : Outport
  wires:
  In1/1 -> LUT 1.10RR/1
  LUT 1.10RR/1 -> Out1/1

== system LUT_liver_pancreas_35/If Action Subsystem6/If Action Subsystem1/If Action Subsystem5/If Action Subsystem3 ==
  In1 : Inport
  Action Port : ActionPort  ActionPortLabel=elseif( u1 >= 1.125)
  LUT 1.13RR : Lookup_n-D  NumberOfTableDimensions=1  BreakpointsForDimension1=[411.4996;552.4418;649.3579;746.0684;842.6134;939.0498;1035.415;1131.731;1228.015;1324.275;1420.517;1516.747;1612.967;1709.18;1805.386;1901.587;1997.784]  Table=[400;500;600;700;800;900;1000;1100;1200;1300;1400;1500;1600;1700;1800;1900;2000]  InternalRulePriority=Speed  RndMeth=Simplest
  Out1 : Outport
  wires:
  In1/1 -> LUT 1.13RR/1
  LUT 1.13RR/1 -> Out1/1

== system LUT_liver_pancreas_35/If Action Subsystem6/If Action Subsystem1/If Action Subsystem5/If Action Subsystem4 ==
  In1 : Inport
  Action Port : ActionPort  ActionPortLabel=elseif( u1 >= 1.135)
  LUT 1.14RR : Lookup_n-D  NumberOfTableDimensions=1  BreakpointsForDimension1=[411.3633;552.1494;648.9508;745.5354;841.9476;938.2465;1034.471;1130.645;1226.784;1322.898;1418.995;1515.077;1611.15;1707.214;1803.272;1899.325;1995.373]  Table=[400;500;600;700;800;900;1000;1100;1200;1300;1400;1500;1600;1700;1800;1900;2000]  InternalRulePriority=Speed  RndMeth=Simplest
  Out1 : Outport
  wires:
  In1/1 -> LUT 1.14RR/1
  LUT 1.14RR/1 -> Out1/1

== system LUT_liver_pancreas_35/If Action Subsystem6/If Action Subsystem1/If Action Subsystem5/If Action Subsystem5 ==
  In1 : Inport
  Action Port : ActionPort  ActionPortLabel=elseif( u1 >= 1.155)
  LUT 1.16RR : Lookup_n-D  NumberOfTableDimensions=1  BreakpointsForDimension1=[411.0969;551.5842;648.165;744.5069;840.6623;936.6953;1032.647;1128.545;1224.404;1320.236;1416.049;1511.846;1607.632;1703.409;1799.179;1894.943;1990.702]  Table=[400;500;600;700;800;900;1000;1100;1200;1300;1400;1500;1600;1700;1800;1900;2000]  InternalRulePriority=Speed  RndMeth=Simplest
  Out1 : Outport
  wires:
  In1/1 -> LUT 1.16RR/1
  LUT 1.16RR/1 -> Out1/1

== system LUT_liver_pancreas_35/If Action Subsystem6/If Action Subsystem1/If Action Subsystem5/If Action Subsystem6 ==
  In1 : Inport
  Action Port : ActionPort  ActionPortLabel=elseif( u1 >= 1.145)
  LUT 1.15RR : Lookup_n-D  NumberOfTableDimensions=1  BreakpointsForDimension1=[411.2291;551.8636;648.5532;745.015;841.2973;937.4618;1033.549;1129.583;1225.581;1321.553;1417.505;1513.444;1609.372;1705.291;1801.204;1897.111;1993.013]  Table=[400;500;600;700;800;900;1000;1100;1200;1300;1400;1500;1600;1700;1800;1900;2000]  InternalRulePriority=Speed  RndMeth=Simplest
  Out1 : Outport
  wires:
  In1/1 -> LUT 1.15RR/1
  LUT 1.15RR/1 -> Out1/1

== system LUT_liver_pancreas_35/If Action Subsystem6/If Action Subsystem1/If Action Subsystem5/If Action Subsystem7 ==
  In1 : Inport
  Action Port : ActionPort  ActionPortLabel=elseif( u1 >= 1.165)
  LUT 1.17RR : Lookup_n-D  NumberOfTableDimensions=1  BreakpointsForDimension1=[410.9666;551.311;647.7859;744.0107;840.0421;935.9464;1031.767;1127.53;1223.254;1318.949;1414.623;1510.282;1605.929;1701.567;1797.197;1892.821;1988.44]  Table=[400;500;600;700;800;900;1000;1100;1200;1300;1400;1500;1600;1700;1800;1900;2000]  InternalRulePriority=Speed  RndMeth=Simplest
  Out1 : Outport
  wires:
  In1/1 -> LUT 1.17RR/1
  LUT 1.17RR/1 -> Out1/1

== system LUT_liver_pancreas_35/If Action Subsystem6/If Action Subsystem1/If Action Subsystem5/If Action Subsystem8 ==
  In1 : Inport
  Action Port : ActionPort  ActionPortLabel=elseif(u1 >= 1.175)
  LUT 1.18RR : Lookup_n-D  NumberOfTableDimensions=1  BreakpointsForDimension1=[410.8384;551.0439;647.4156;743.5262;839.4363;935.2146;1030.906;1126.538;1222.128;1317.689;1413.228;1508.751;1604.262;1699.763;1795.256;1890.743;1986.224]  Table=[400;500;600;700;800;900;1000;1100;1200;1300;1400;1500;1600;1700;1800;1900;2000]  InternalRulePriority=Speed  RndMeth=Simplest
  Out1 : Outport
  wires:
  In1/1 -> LUT 1.18RR/1
  LUT 1.18RR/1 -> Out1/1

== system LUT_liver_pancreas_35/If Action Subsystem6/If Action Subsystem1/If Action Subsystem5/If Action Subsystem9 ==
  In1 : Inport
  Action Port : ActionPort  ActionPortLabel=if(u1 >= 1.185)
  LUT 1.19RR : Lookup_n-D  NumberOfTableDimensions=1  BreakpointsForDimension1=[410.712;550.7826;647.0538;743.0529;838.8444;934.4994;1030.064;1125.567;1221.027;1316.457;1411.864;1507.253;1602.63;1697.997;1793.355;1888.707;1984.053]  Table=[400;500;600;700;800;900;1000;1100;1200;1300;1400;1500;1600;1700;1800;1900;2000]  InternalRulePriority=Speed  RndMeth=Simplest
  Out1 : Outport
  wires:
  In1/1 -> LUT 1.19RR/1
  LUT 1.19RR/1 -> Out1/1

== system LUT_liver_pancreas_35/If Action Subsystem6/If Action Subsystem1/If Action Subsystem6/If Action Subsystem1 ==
  In1 : Inport
  Action Port : ActionPort  ActionPortLabel=elseif( u1 >= 1.015)
  LUT 1.02RR : Lookup_n-D  NumberOfTableDimensions=1  BreakpointsForDimension1=[413.1508;556.151;654.5592;752.8828;851.1156;949.2882;1047.422;1145.531;1243.622;1341.703;1439.775;1537.841;1635.903;1733.962;1832.017;1930.069;2028.117]  Table=[400;500;600;700;800;900;1000;1100;1200;1300;1400;1500;1600;1700;1800;1900;2000]  InternalRulePriority=Speed  RndMeth=Simplest
  Out1 : Outport
  wires:
  In1/1 -> LUT 1.02RR/1
  LUT 1.02RR/1 -> Out1/1

== system LUT_liver_pancreas_35/If Action Subsystem6/If Action Subsystem1/If Action Subsystem6/If Action Subsystem10 ==
  In1 : Inport
  Action Port : ActionPort  ActionPortLabel=elseif( u1 >= 1.005)
  LUT 1.01RR : Lookup_n-D  NumberOfTableDimensions=1  BreakpointsForDimension1=[413.3161547;556.5392657;655.1070022;753.6009136;852.0106415;950.3643269;1048.682093;1146.976569;1245.255617;1343.524203;1441.785506;1540.041581;1638.293731;1736.542717;1834.788833;1933.03182;2031.27041]  Table=[400;500;600;700;800;900;1000;1100;1200;1300;1400;1500;1600;1700;1800;1900;2000]  InternalRulePriority=Speed  RndMeth=Simplest
  Out1 : Outport
  wires:
  In1/1 -> LUT 1.01RR/1
  LUT 1.01RR/1 -> Out1/1

== system LUT_liver_pancreas_35/If Action Subsystem6/If Action Subsystem1/If Action Subsystem6/If Action Subsystem2 ==
  In1 : Inport
  Action Port : ActionPort  ActionPortLabel=else
  LUT 1.00RR : Lookup_n-D  NumberOfTableDimensions=1  BreakpointsForDimension1=[413.4843;556.9372;655.669;754.3378;852.9289;951.4681;1049.974;1148.459;1246.93;1345.391;1443.846;1542.296;1640.743;1739.186;1837.627;1936.065;2034.499]  Table=[400;500;600;700;800;900;1000;1100;1200;1300;1400;1500;1600;1700;1800;1900;2000]  InternalRulePriority=Speed  RndMeth=Simplest
  Out1 : Outport
  wires:
  In1/1 -> LUT 1.00RR/1
  LUT 1.00RR/1 -> Out1/1
